simulink model "simura"  (R2018a)
settings: Solver=VariableStepAuto  StartTime=0.0  StopTime=10  MaxStep=0.01  RelTol=1e-4  EnableMultiTasking=on
settings Model: Creator=user  LastModifiedBy=user
settings DataIOCC: LimitDataPoints=on  SaveOutput=off  SaveTime=off
settings OptimizationCC: ExpressionDepthLimit=2147483647  LifeSpan=1
settings DebuggingCC: UnderspecifiedInitializationDetection=Classic  MergeDetectMultiDrivingBlocksExec=none  FcnCallInpInsideContextMsg=warning  AllowSymbolicDim=off  StateNameClashWarn=warning  SFUnexpectedBacktrackingDiag=warning  SFNoUnconditionalDefaultTransitionDiag=warning  SFExecutionAtInitializationDiag=none
settings CodeAppCC: StateflowObjectComments=on
settings GRTTargetCC: TargetLangStandard=C89/C90 (ANSI)  GeneratePreprocessorConditionals=Disable all  CombineOutputUpdateFcns=off  GRTInterface=on

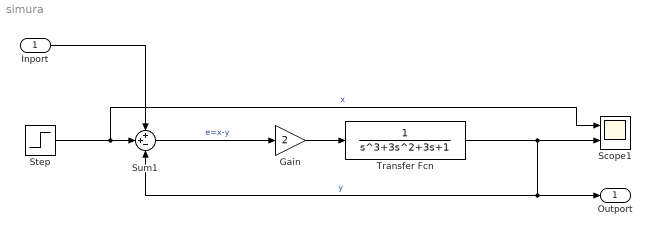
== system simura ==
  Inport : Inport  Description=Wywolanie funkcji w Command Window
      settings: AttributesFormatString=Inport
  Gain : Gain  Description=Wzmocnienie sygnalu  Gain=2
      settings: AttributesFormatString=Gain
  Scope1 : Scope  NumInputPorts=2
      settings: Description=Przebiegi x(t), y(t)  AttributesFormatString=Scope
  Step : Step  Description=Skok jednostkowy  SampleTime=0
      settings: AttributesFormatString=Step
  Sum1 : Sum  Description=Suma algebraiczna sygnalow  Inputs=++-
      settings: AttributesFormatString=Sum
  Transfer Fcn : TransferFcn  Description=G(s)=L(s)/M(s), L-wsp. licznika, M-wsp.mainownika  Denominator=[1 3 3 1]
      settings: AttributesFormatString=Transfer Fcn
  Outport : Outport  Description=Wyniki funkcji Matlaba w Command Window
      settings: AttributesFormatString=Outport
  wires:
  Step/1 -> Sum1/2, Scope1/1  "x"
  Sum1/1 -> Gain/1  "e=x-y"
  Gain/1 -> Transfer Fcn/1
  Transfer Fcn/1 -> Scope1/2, Sum1/3, Outport/1  "y"
  Inport/1 -> Sum1/1
